simulink model "vel_pose_connect_sl"  (R2018b)
settings: Solver=VariableStepAuto  StartTime=0.0  StopTime=inf  RelTol=1e-3
undefined symbols (not defined in the file): Angle, Brakepedal, Drivemode, Drivepedal, Gearshift, Header, Lamp, Light, Speed, Steeringmode, Tm, Twist
libraries: robotlib x19
settings Model: Creator=handai  LastModifiedBy=handai

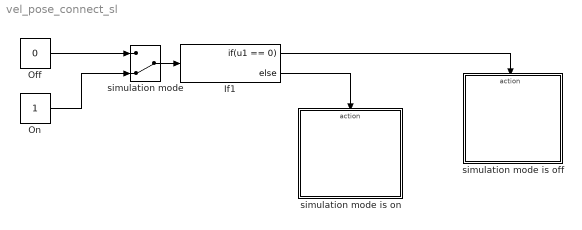
== system vel_pose_connect_sl ==
  If1 : If  IfExpression=u1 == 0
  Off : Constant  Value=0
  On : Constant
  simulation mode : ManualSwitch  CurrentSetting=0
  simulation mode is off : Subsystem  TreatAsAtomicUnit=on
  simulation mode is on : Subsystem  TreatAsAtomicUnit=on
  wires:
  Off/1 -> simulation mode/1
  On/1 -> simulation mode/2
  simulation mode/1 -> If1/1
  If1/1 -> simulation mode is off/Action
  If1/2 -> simulation mode is on/Action

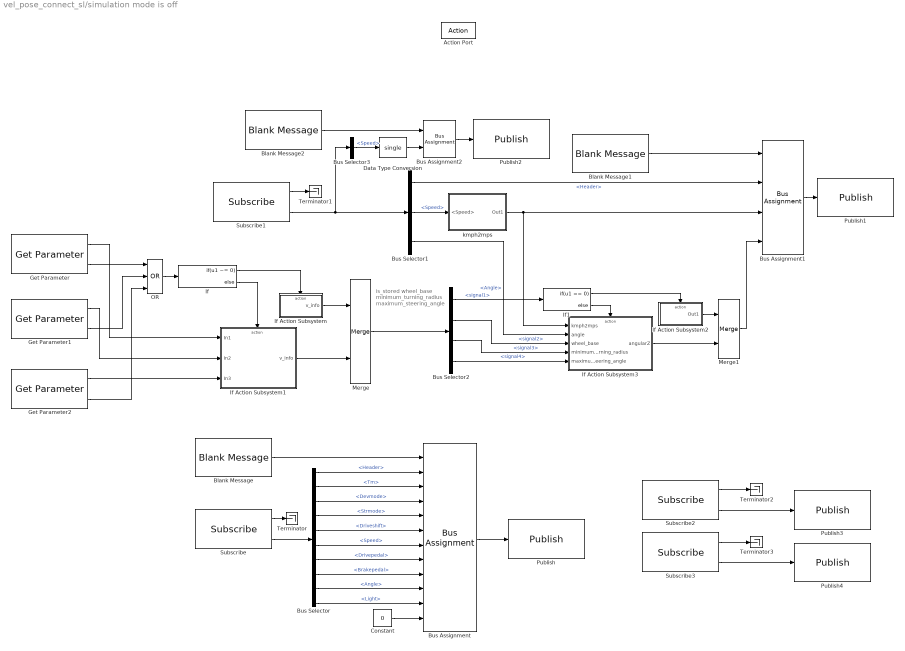
== system vel_pose_connect_sl/simulation mode is off ==
  note: is_stored
      | wheel_base
      | minimum_turning_radius
      | maximum_steering_angle
  Action Port : ActionPort  ActionType=then
  Blank Message : robotlib/Blank Message  messageClass=Message  entityType=autoware_msgs/VehicleStatus  messageType=autoware_msgs/VehicleStatus  SampleTime=inf
      settings: SourceProductBaseCode=RO
  Blank Message1 : robotlib/Blank Message  messageClass=Message  entityType=geometry_msgs/TwistStamped  messageType=geometry_msgs/TwistStamped  SampleTime=inf
      settings: SourceProductBaseCode=RO
  Blank Message2 : robotlib/Blank Message  messageClass=Message  entityType=std_msgs/Float32  messageType=std_msgs/Float32  SampleTime=inf
      settings: SourceProductBaseCode=RO
  Bus Assignment : BusAssignment  AssignedSignals=Header,Tm,Drivemode,Steeringmode,Gearshift,Speed,Drivepedal,Brakepedal,Angle,Light,Lamp
  Bus Assignment1 : BusAssignment  AssignedSignals=Header,Twist.Linear.X,Twist.Angular.Z
  Bus Assignment2 : BusAssignment  AssignedSignals=Data
  Bus Selector : BusSelector  OutputSignals=Header,Tm,Devmode,Strmode,Driveshift,Speed,Drivepedal,Brakepedal,Angle,Light
  Bus Selector1 : BusSelector  OutputSignals=Header,Speed,Angle
  Bus Selector2 : BusSelector  OutputSignals=signal1,signal2,signal3,signal4
  Bus Selector3 : BusSelector  OutputSignals=Speed
  Constant : Constant  Value=0  OutDataTypeStr=int32
  Data Type Conversion : DataTypeConversion  OutDataTypeStr=single
  Get Parameter : robotlib/Get Parameter  ParameterSource=Specify your own  ParameterName=/vehicle_info/wheel_base  ParameterType=double  ParameterMaxArrayLength=16  ParameterInitialValue=0.0  SampleTime=-1  ShowErrorCodeOutput=on  ModelName=vel_pose_connect_sl  BlockId=ParamGet_vel_pose_connect_sl_17
      settings: SourceProductName=Robotics System Toolbox  SourceProductBaseCode=RO
  Get Parameter1 : robotlib/Get Parameter  ParameterSource=Specify your own  ParameterName=/vehicle_info/minimum_turning_radius  ParameterType=double  ParameterMaxArrayLength=16  ParameterInitialValue=0.0  SampleTime=-1  ShowErrorCodeOutput=on  ModelName=vel_pose_connect_sl  BlockId=ParamGet_vel_pose_connect_sl_18
      settings: SourceProductName=Robotics System Toolbox  SourceProductBaseCode=RO
  Get Parameter2 : robotlib/Get Parameter  ParameterSource=Specify your own  ParameterName=/vehicle_info/maximum_steering_angle  ParameterType=double  ParameterMaxArrayLength=16  ParameterInitialValue=0.0  SampleTime=-1  ShowErrorCodeOutput=on  ModelName=vel_pose_connect_sl  BlockId=ParamGet_vel_pose_connect_sl_19
      settings: SourceProductName=Robotics System Toolbox  SourceProductBaseCode=RO
  If : If  IfExpression=u1 ~= 0
  If Action Subsystem : Subsystem  TreatAsAtomicUnit=on
  If Action Subsystem1 : Subsystem  TreatAsAtomicUnit=on
  If Action Subsystem2 : Subsystem  TreatAsAtomicUnit=on
  If Action Subsystem3 : Subsystem  TreatAsAtomicUnit=on
  If1 : If  IfExpression=u1 == 0
  Merge : Merge
  Merge1 : Merge
  OR : Logic  Operator=OR  Inputs=3  IconShape=distinctive  AllPortsSameDT=off  OutDataTypeStr=boolean
  Publish : robotlib/Publish  topicSource=Specify your own  topic=/vehicle_status  messageType=autoware_msgs/VehicleStatus  messageQueueLength=1
      settings: SourceProductBaseCode=RO
  Publish1 : robotlib/Publish  topicSource=Specify your own  topic=/can_velocity  messageType=geometry_msgs/TwistStamped  messageQueueLength=1
      settings: SourceProductBaseCode=RO
  Publish2 : robotlib/Publish  topicSource=Specify your own  topic=/linear_velocity_viz  messageType=std_msgs/Float32  messageQueueLength=1
      settings: SourceProductBaseCode=RO
  Publish3 : robotlib/Publish  topicSource=Specify your own  topic=/current_pose  messageType=geometry_msgs/PoseStamped  messageQueueLength=1
      settings: SourceProductBaseCode=RO
  Publish4 : robotlib/Publish  topicSource=Specify your own  topic=/current_velocity  messageType=geometry_msgs/TwistStamped  messageQueueLength=1
      settings: SourceProductBaseCode=RO
  Subscribe : robotlib/Subscribe  topicSource=Specify your own  topic=/can_info  messageType=autoware_msgs/CanInfo  sampleTime=-1  messageQueueLength=1
      settings: SourceProductBaseCode=RO
  Subscribe1 : robotlib/Subscribe  topicSource=Specify your own  topic=/vehicle_status  messageType=autoware_msgs/VehicleStatus  sampleTime=-1  messageQueueLength=1
      settings: SourceProductBaseCode=RO
  Subscribe2 : robotlib/Subscribe  topicSource=Specify your own  topic=/ndt_pose  messageType=geometry_msgs/PoseStamped  sampleTime=-1  messageQueueLength=1
      settings: SourceProductBaseCode=RO
  Subscribe3 : robotlib/Subscribe  topicSource=Specify your own  topic=/estimate_twist  messageType=geometry_msgs/TwistStamped  sampleTime=-1  messageQueueLength=1
      settings: SourceProductBaseCode=RO
  Terminator{,1..3} (4 alike) : Terminator
  kmph2mps : Subsystem
  wires:
  Get Parameter2/2 -> OR/3
  If/2 -> If Action Subsystem1/Action
  Get Parameter1/2 -> OR/2
  OR/1 -> If/1
  Get Parameter/2 -> OR/1
  If/1 -> If Action Subsystem/Action
  Get Parameter/1 -> If Action Subsystem1/1(In1)
  Get Parameter1/1 -> If Action Subsystem1/2(In2)
  Get Parameter2/1 -> If Action Subsystem1/3(In3)
  If Action Subsystem/1(v_info) -> Merge/1
  If Action Subsystem1/1(v_info) -> Merge/2
  Subscribe/2 -> Bus Selector/1
  Blank Message/1 -> Bus Assignment/1
  Bus Selector/1 -> Bus Assignment/2  "<Header>"
  Bus Selector/2 -> Bus Assignment/3  "<Tm>"
  Bus Selector/3 -> Bus Assignment/4  "<Devmode>"
  Bus Selector/4 -> Bus Assignment/5  "<Strmode>"
  Bus Selector/5 -> Bus Assignment/6  "<Driveshift>"
  Bus Selector/6 -> Bus Assignment/7  "<Speed>"
  Bus Selector/7 -> Bus Assignment/8  "<Drivepedal>"
  Bus Selector/8 -> Bus Assignment/9  "<Brakepedal>"
  Bus Selector/9 -> Bus Assignment/10  "<Angle>"
  Bus Selector/10 -> Bus Assignment/11  "<Light>"
  Bus Assignment/1 -> Publish/1
  Constant/1 -> Bus Assignment/12
  Subscribe/1 -> Terminator/1
  Subscribe1/2 -> Bus Selector3/1, Bus Selector1/1
  Bus Selector1/2 -> kmph2mps/1(<Speed>)  "<Speed>"
  Blank Message1/1 -> Bus Assignment1/1
  kmph2mps/1(Out1) -> Bus Assignment1/3, If Action Subsystem3/1(kmph2mps)
  Bus Selector1/1 -> Bus Assignment1/2  "<Header>"
  Bus Selector1/3 -> If Action Subsystem3/2(angle)  "<Angle>"
  Merge/1 -> Bus Selector2/1
  Bus Selector2/1 -> If1/1  "<signal1>"
  If1/1 -> If Action Subsystem2/Action
  If1/2 -> If Action Subsystem3/Action
  Bus Selector2/4 -> If Action Subsystem3/5(maximum_steering_angle)  "<signal4>"
  Bus Selector2/3 -> If Action Subsystem3/4(minimum_turning_radius)  "<signal3>"
  Bus Selector2/2 -> If Action Subsystem3/3(wheel_base)  "<signal2>"
  If Action Subsystem3/1(angularZ) -> Merge1/2
  If Action Subsystem2/1(Out1) -> Merge1/1
  Merge1/1 -> Bus Assignment1/4
  Bus Assignment1/1 -> Publish1/1
  Subscribe1/1 -> Terminator1/1
  Bus Selector3/1 -> Data Type Conversion/1  "<Speed>"
  Blank Message2/1 -> Bus Assignment2/1
  Bus Assignment2/1 -> Publish2/1
  Data Type Conversion/1 -> Bus Assignment2/2
  Subscribe2/2 -> Publish3/1
  Subscribe3/2 -> Publish4/1
  Subscribe2/1 -> Terminator2/1
  Subscribe3/1 -> Terminator3/1

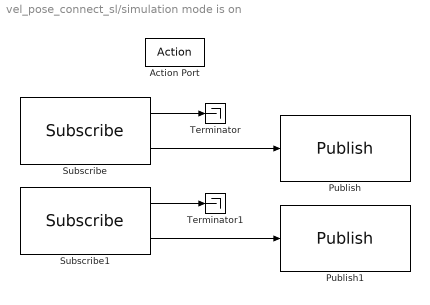
== system vel_pose_connect_sl/simulation mode is on ==
  Action Port : ActionPort  ActionType=else
  Publish : robotlib/Publish  topicSource=Specify your own  topic=/current_pose  messageType=geometry_msgs/PoseStamped  messageQueueLength=1
      settings: SourceProductBaseCode=RO
  Publish1 : robotlib/Publish  topicSource=Specify your own  topic=/current_velocity  messageType=geometry_msgs/TwistStamped  messageQueueLength=1
      settings: SourceProductBaseCode=RO
  Subscribe : robotlib/Subscribe  topicSource=Specify your own  topic=/sim_pose  messageType=geometry_msgs/PoseStamped  sampleTime=-1  messageQueueLength=1
      settings: SourceProductBaseCode=RO
  Subscribe1 : robotlib/Subscribe  topicSource=Specify your own  topic=/sim_velocity  messageType=geometry_msgs/TwistStamped  sampleTime=-1  messageQueueLength=1
      settings: SourceProductBaseCode=RO
  Terminator : Terminator
  Terminator1 : Terminator
  wires:
  Subscribe/2 -> Publish/1
  Subscribe1/2 -> Publish1/1
  Subscribe/1 -> Terminator/1
  Subscribe1/1 -> Terminator1/1

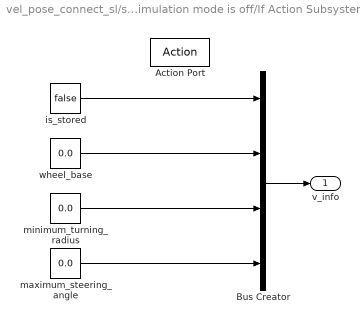
== system vel_pose_connect_sl/simulation mode is off/If Action Subsystem ==
  Action Port : ActionPort  ActionType=then
  Bus Creator : BusCreator  Inputs=4
  is_stored : Constant  Value=false  OutDataTypeStr=boolean
  maximum_steering_angle : Constant  Value=0.0  OutDataTypeStr=double
  minimum_turning_radius : Constant  Value=0.0  OutDataTypeStr=double
  wheel_base : Constant  Value=0.0  OutDataTypeStr=double
  v_info : Outport
  wires:
  is_stored/1 -> Bus Creator/1
  wheel_base/1 -> Bus Creator/2
  minimum_turning_radius/1 -> Bus Creator/3
  maximum_steering_angle/1 -> Bus Creator/4
  Bus Creator/1 -> v_info/1

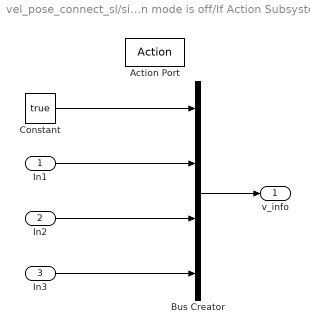
== system vel_pose_connect_sl/simulation mode is off/If Action Subsystem1 ==
  In1 : Inport
  In2 : Inport  Port=2
  In3 : Inport  Port=3
  Action Port : ActionPort  ActionType=else
  Bus Creator : BusCreator  Inputs=4
  Constant : Constant  Value=true  OutDataTypeStr=boolean
  v_info : Outport
  wires:
  Constant/1 -> Bus Creator/1
  In1/1 -> Bus Creator/2
  In2/1 -> Bus Creator/3
  In3/1 -> Bus Creator/4
  Bus Creator/1 -> v_info/1

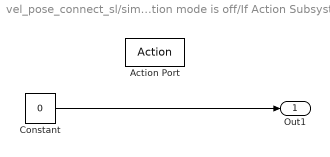
== system vel_pose_connect_sl/simulation mode is off/If Action Subsystem2 ==
  Action Port : ActionPort  ActionType=then
  Constant : Constant  Value=0  OutDataTypeStr=double
  Out1 : Outport
  wires:
  Constant/1 -> Out1/1

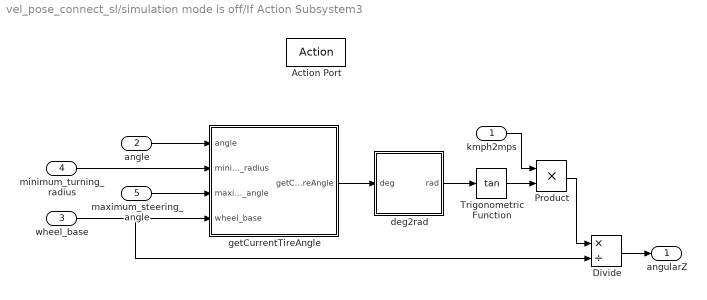
== system vel_pose_connect_sl/simulation mode is off/If Action Subsystem3 ==
  kmph2mps : Inport
  angle : Inport  Port=2
  wheel_base : Inport  Port=3
  minimum_turning_radius : Inport  Port=4
  maximum_steering_angle : Inport  Port=5
  Action Port : ActionPort  ActionType=else
  Divide : Product  Inputs=*/
  Product : Product
  Trigonometric Function : Trigonometry  Operator=tan
  deg2rad : Subsystem
  getCurrentTireAngle : Subsystem
  angularZ : Outport
  wires:
  kmph2mps/1 -> Product/1
  angle/1 -> getCurrentTireAngle/1(angle)
  wheel_base/1 -> getCurrentTireAngle/4(wheel_base), Divide/2
  minimum_turning_radius/1 -> getCurrentTireAngle/2(minimum_turning_radius)
  maximum_steering_angle/1 -> getCurrentTireAngle/3(maximum_steering_angle)
  getCurrentTireAngle/1(getCurrentTireAngle) -> deg2rad/1(deg)
  deg2rad/1(rad) -> Trigonometric Function/1
  Trigonometric Function/1 -> Product/2
  Product/1 -> Divide/1
  Divide/1 -> angularZ/1

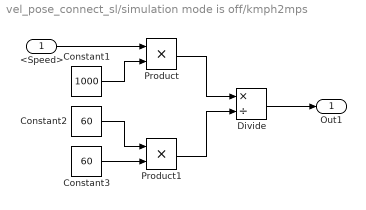
== system vel_pose_connect_sl/simulation mode is off/kmph2mps ==
  <Speed> : Inport
  Constant1 : Constant  Value=1000
  Constant2 : Constant  Value=60
  Constant3 : Constant  Value=60
  Divide : Product  Inputs=*/
  Product : Product
  Product1 : Product
  Out1 : Outport
  wires:
  Constant1/1 -> Product/2
  Constant2/1 -> Product1/1
  Constant3/1 -> Product1/2
  <Speed>/1 -> Product/1
  Divide/1 -> Out1/1
  Product/1 -> Divide/1
  Product1/1 -> Divide/2

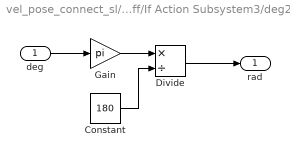
== system vel_pose_connect_sl/simulation mode is off/If Action Subsystem3/deg2rad ==
  deg : Inport
  Constant : Constant  Value=180
  Divide : Product  Inputs=*/
  Gain : Gain  Gain=pi
  rad : Outport
  wires:
  Constant/1 -> Divide/2
  deg/1 -> Gain/1
  Gain/1 -> Divide/1
  Divide/1 -> rad/1

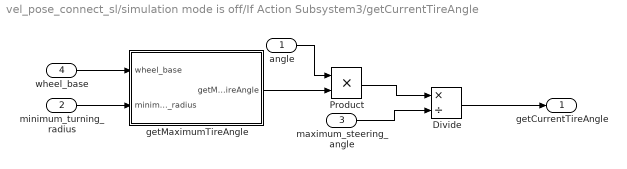
== system vel_pose_connect_sl/simulation mode is off/If Action Subsystem3/getCurrentTireAngle ==
  angle : Inport
  minimum_turning_radius : Inport  Port=2
  maximum_steering_angle : Inport  Port=3
  wheel_base : Inport  Port=4
  Divide : Product  Inputs=*/
  Product : Product
  getMaximumTireAngle : Subsystem
  getCurrentTireAngle : Outport
  wires:
  Product/1 -> Divide/1
  getMaximumTireAngle/1(getMaximumTireAngle) -> Product/2
  minimum_turning_radius/1 -> getMaximumTireAngle/2(minimum_turning_radius)
  wheel_base/1 -> getMaximumTireAngle/1(wheel_base)
  Divide/1 -> getCurrentTireAngle/1
  angle/1 -> Product/1
  maximum_steering_angle/1 -> Divide/2

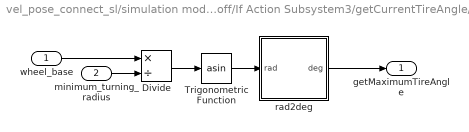
== system vel_pose_connect_sl/simulation mode is off/If Action Subsystem3/getCurrentTireAngle/getMaximumTireAngle ==
  wheel_base : Inport
  minimum_turning_radius : Inport  Port=2
  Divide : Product  Inputs=*/
  Trigonometric Function : Trigonometry  Operator=asin
  rad2deg : Subsystem
  getMaximumTireAngle : Outport
  wires:
  wheel_base/1 -> Divide/1
  Trigonometric Function/1 -> rad2deg/1(rad)
  minimum_turning_radius/1 -> Divide/2
  Divide/1 -> Trigonometric Function/1
  rad2deg/1(deg) -> getMaximumTireAngle/1

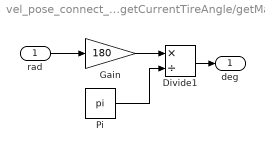
== system vel_pose_connect_sl/simulation mode is off/If Action Subsystem3/getCurrentTireAngle/getMaximumTireAngle/rad2deg ==
  rad : Inport
  Divide1 : Product  Inputs=*/
  Gain : Gain  Gain=180
  Pi : Constant  Value=pi  OutDataTypeStr=Inherit: Inherit via back propagation
  deg : Outport
  wires:
  Pi/1 -> Divide1/2
  Gain/1 -> Divide1/1
  rad/1 -> Gain/1
  Divide1/1 -> deg/1
